simulink model "model432"  (R2014a)
settings: Solver=ode1  StartTime=0.0  StopTime=inf  FixedStep=0.002  RelTol=1e-3
PostLoadFcn:
  | qc_set_target_type(getConfigSet(bdroot, 'QUARC Default Target Configuration'));
values from neighbouring files (symbols this model uses):
  A_o = [0 1 0 0 0 0; 0 0 0 0 0 0; 0 0 0 1 0 0; 0 0 0 0 0 0; 0 0 0 0 0 1; K_3 0 0 0 0 0]    [Full_code.m]    (also in code421.m; code422.m; code431.m; code432.m)
  B_o = [0 0; 0 K_1; 0 0; K_2 0; 0 0; 0 0]    [Full_code.m]    (also in code421.m; code422.m; code431.m; code432.m)
  C_o = [1 0 0 0 0 0; 0 0 1 0 0 0; 0 0 0 0 1 0]    [Full_code.m]    (also in code421.m; code422.m; code431.m = [0 0 1 0 0 0; 0 0 0 0 1 0]; code432.m = [0 0 1 0 0 0; 0 0 0 0 1 0])
  Joystick_gain_x = 1    [Full_code.m]    (also in code13.m; code14.m; code21.m; code22.m)
  Joystick_gain_y = -1    [Full_code.m]    (also in code13.m; code14.m; code21.m; code22.m)
  K = lqr(A,B,Q,R)    [Full_code.m]    (also in code32.m; code33.m; code421.m; code422.m)
  L_o = place(transpose(A_o), transpose(C_o),poles).'    [Full_code.m]    (also in code421.m; code422.m; code431.m = place(transpose(A_o), transpose(C_o), poles).'; code432.m = place(transpose(A_o), transpose(C_o), poles).')
  P = [0 9.999999999999998;9.549869109050656 0]    [Full_code.m]    (also in code32.m = inv(C*inv(-A+B*K)*B); code33.m; code421.m = inv(C*inv(-A+B*K)*B); code422.m)
undefined symbols (not defined in the file or in its folder): HIL, qc_get_step_size
libraries: simulink_extras x6, quarc_library x4
settings Model: SimulationMode=external  ExtModeTrigDuration=5000  Creator=Rchan  LastModifiedBy=mortejan
settings SolverCC: PositivePriorityOrder=on
settings DataIOCC: SignalLoggingSaveFormat=ModelDataLogs
settings OptimizationCC: ExpressionDepthLimit=2147483647  InitFltsAndDblsToZero=on
settings DebuggingCC: SaveWithParameterizedLinksMsg=none  UnderspecifiedInitializationDetection=Classic  MultiTaskDSMMsg=warning  MultiTaskCondExecSysMsg=none  FcnCallInpInsideContextMsg=UseLocalSettings  StateNameClashWarn=warning
settings RTWCC: SystemTargetFile=quarc_win64.tlc  TemplateMakefile=quarc_default_tmf  Description=QUARC Win64 Target  ProcessScript=quarc_win64_make_rtw_hook
settings STFCustomTargetCC: CPPClassGenCompliant=on
settings GRTTargetCC: ParMdlRefBuildCompliant=off  CompOptLevelCompliant=off  CombineOutputUpdateFcns=off  MatFileLogging=off  GRTInterface=on  ExtMode=on  ExtModeMexFile=quarc_comm

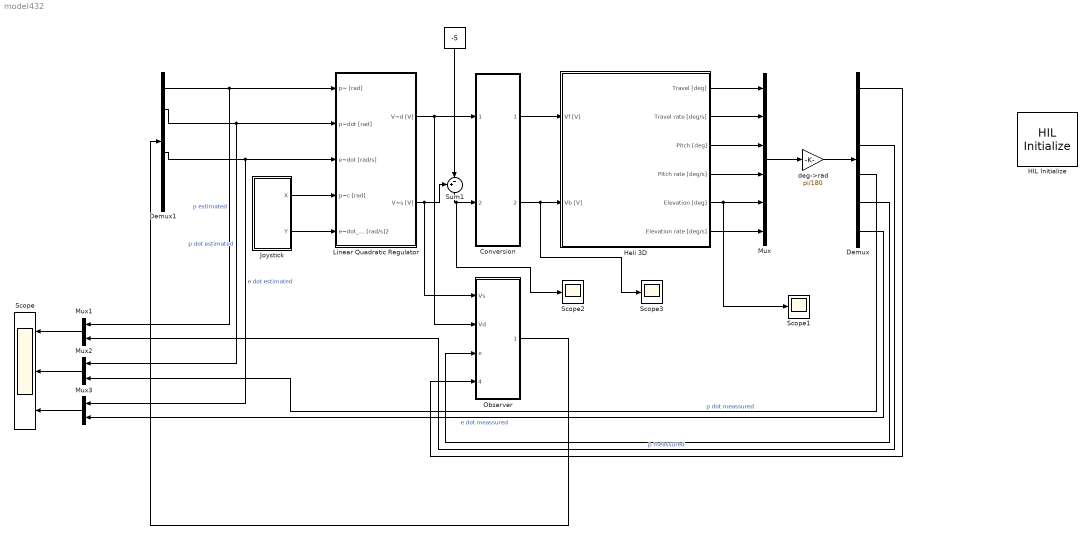
== system model432 ==
  " " : Constant  Value=-5
  Conversion : Subsystem
  Demux : Demux  Outputs=6
  Demux1 : Demux  Outputs=6
  HIL Initialize : quarc_library/Data Acquisition/Generic/Configuration/HIL Initialize  Priority=-99  object_name=HIL-1  board_type=q8_usb  board_number=0  board_options=update_rate=normal;decimation=1  exclusive=off  active=off  hardware_clocks=[0:2]  clock_modes=[]  initial_clock_frequencies=[]  set_clock_params_at_start=off  set_clock_params_at_switch_in=off  set_clock_frequencies_at_start=off  set_clock_frequencies_at_switch_in=off  analog_input_channels=[0:7]  analog_input_maximums=10  analog_input_minimums=-10  set_analog_input_params_at_start=on  set_analog_input_params_at_switch_in=off  analog_output_channels=[0:7]  analog_output_maximums=10  analog_output_minimums=-10  initial_analog_outputs=[0]  final_analog_outputs=[0]  watchdog_analog_outputs=0  set_analog_output_params_at_start=on  set_analog_output_params_at_switch_in=off  set_analog_outputs_at_start=on  set_analog_outputs_at_switch_in=off  set_analog_outputs_at_terminate=on  set_analog_outputs_at_switch_out=off  set_analog_outputs_on_watchdog=off  digital_input_channels=[]  digital_output_channels=[]  digital_output_configuration=[]  initial_digital_outputs=[1]  final_digital_outputs=[1]  watchdog_digital_outputs=[1]  set_digital_output_params_at_start=off  set_digital_output_params_at_switch_in=off  set_digital_outputs_at_start=on  set_digital_outputs_at_switch_in=off  set_digital_outputs_at_terminate=on  set_digital_outputs_at_switch_out=off  set_digital_outputs_on_watchdog=off  encoder_channels=[0:7]  quadrature=[4]  encoder_filter_frequency=[]  initial_encoder_counts=[0]  set_encoder_params_at_start=on  set_encoder_params_at_switch_in=off  set_encoder_counts_at_start=on  set_encoder_counts_at_switch_in=off  pwm_channels=[0:7]  pwm_modes=0  pwm_frequency=99.532799999999995e6/4095  pwm_configuration=[0]  pwm_alignment=[0]  pwm_polarity=[1]  pwm_leading_deadband=[0]  pwm_trailing_deadband=[0]  initial_pwm_outputs=[0]  final_pwm_outputs=[0]  watchdog_pwm_outputs=[0]  set_pwm_params_at_start=on  set_pwm_params_at_switch_in=off  set_pwm_outputs_at_start=on  set_pwm_outputs_at_switch_in=off  set_pwm_outputs_at_terminate=on  set_pwm_outputs_at_switch_out=off  set_pwm_outputs_on_watchdog=off  other_output_channels=[]  initial_other_outputs=[]  final_other_outputs=[]  watchdog_other_outputs=[]  set_other_outputs_at_start=off  set_other_outputs_at_switch_in=off  set_other_outputs_at_terminate=off  set_other_outputs_at_switch_out=off  set_other_outputs_on_watchdog=off
  Heli 3D : Subsystem
  Joystick : Subsystem
  Linear Quadratic Regulator : Subsystem
  Mux : Mux  Inputs=6
  Mux1 : Mux  Inputs=2
  Mux2 : Mux  Inputs=2
  Mux3 : Mux  Inputs=2
  Observer : Subsystem
  Scope : Scope  NumInputPorts=3
      settings: ShowLegends=on  YMin=-0.4~-1.5~-0.6  YMax=1~1.5~0.6  SaveName=ScopeData3  MaxDataPoints=10000
  Scope1 : Scope
      settings: SaveName=ScopeData4
  Scope2 : Scope
      settings: SaveName=ScopeData6
  Scope3 : Scope
      settings: SaveName=ScopeData14
  Sum1 : Sum  Inputs=+-|
  deg->rad : Gain  Gain=pi/180
  wires:
  Conversion/2(Vb [V]) -> Scope3/1, Heli 3D/2(Vb [V])
  Conversion/1(Vf [V]) -> Heli 3D/1(Vf [V])
  Heli 3D/1(Travel [deg]) -> Mux/1
  Heli 3D/2(Travel rate [deg/s]) -> Mux/2
  Heli 3D/3(Pitch [deg]) -> Mux/3
  Heli 3D/4(Pitch rate [deg/s]) -> Mux/4
  Heli 3D/5(Elevation [deg]) -> Scope1/1, Mux/5
  Heli 3D/6(Elevation rate [deg/s]) -> Mux/6
  Mux/1 -> deg->rad/1
  deg->rad/1 -> Demux/1
  Joystick/1(X) -> Linear Quadratic Regulator/4(p~c [rad])
  Joystick/2(Y) -> Linear Quadratic Regulator/5(e~dot_c [rad/s]2)
  Linear Quadratic Regulator/1(V~d [V]) -> Observer/2(Vd), Conversion/1(Vd [V])
  Linear Quadratic Regulator/2(V~s [V]) -> Observer/1(Vs), Sum1/1
  Demux/5 -> Observer/3(e)
  Demux/1 -> Observer/4(lambda)
  Observer/1(x_obs) -> Demux1/1
  Demux1/1 -> Mux1/1, Linear Quadratic Regulator/1(p~ [rad])  "p estimated"
  Demux1/2 -> Mux2/1, Linear Quadratic Regulator/2(p~dot [rad])  "p dot estimated"
  Demux1/4 -> Mux3/1, Linear Quadratic Regulator/3(e~dot [rad/s])  "e dot estimated"
  Demux/3 -> Mux1/2  "p meassured"
  Mux1/1 -> Scope/1
  Mux3/1 -> Scope/3
  Mux2/1 -> Scope/2
  Demux/4 -> Mux2/2  "p dot meassured"
  Demux/6 -> Mux3/2  "e dot meassured"
  " "/1 -> Sum1/2
  Sum1/1 -> Scope2/1, Conversion/2(Vs [V])

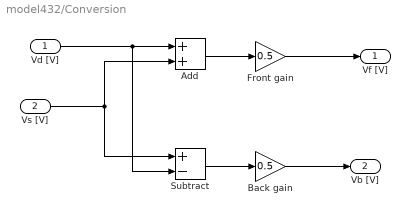
== system model432/Conversion ==
  Vd [V] : Inport
  Vs [V] : Inport  Port=2
  Add : Sum
  Back gain : Gain  Gain=0.5
  Front gain : Gain  Gain=0.5
  Subtract : Sum  Inputs=+-
  Vf [V] : Outport
  Vb [V] : Outport  Port=2
  wires:
  Vd [V]/1 -> Subtract/2, Add/1
  Vs [V]/1 -> Subtract/1, Add/2
  Subtract/1 -> Back gain/1
  Back gain/1 -> Vb [V]/1
  Add/1 -> Front gain/1
  Front gain/1 -> Vf [V]/1

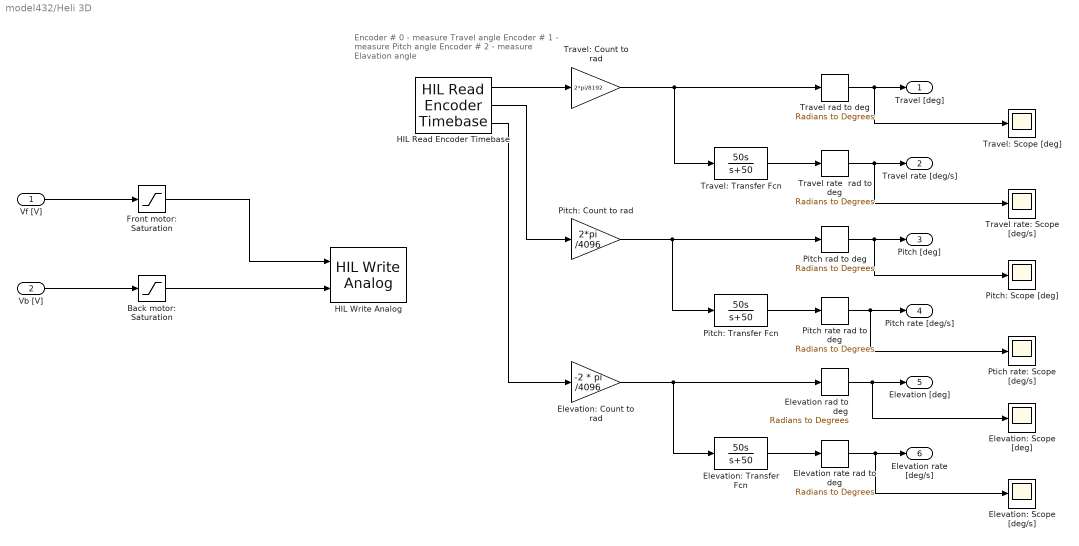
== system model432/Heli 3D ==
  note: Encoder # 0 - measure Travel angle
      | Encoder # 1 - measure Pitch angle
      | Encoder # 2 - measure Elavation angle
  Vf [V] : Inport
  Vb [V] : Inport  Port=2
  Back motor: Saturation : Saturate  UpperLimit=5  LowerLimit=-5
  Elevation rad to deg : simulink_extras/Transformations/Radians to Degrees
  Elevation rate rad to deg : simulink_extras/Transformations/Radians to Degrees
  Elevation: Count to rad : Gain  Gain=-2 * pi /4096
  Elevation: Scope [deg/s] : Scope
      settings: YMin=-15  YMax=15  SaveName=ScopeData13
  Elevation: Scope [deg] : Scope
      settings: YMin=-15  YMax=15  SaveName=ScopeData12
  Elevation: Transfer Fcn : TransferFcn  Numerator=[50 0]  Denominator=[1 50]
  Front motor: Saturation : Saturate  UpperLimit=5  LowerLimit=-5
  HIL Read Encoder Timebase : quarc_library/Data Acquisition/Generic/Timebases/HIL Read Encoder Timebase  object_name=HIL-1  clock=0  channels=[0:2]  samples_in_buffer=max(ceil(1/qc_get_step_size), 1)  active=on  vector_output=off  data_type_mode=Inherit via back propagation  data_type=double
  HIL Write Analog : quarc_library/Data Acquisition/Generic/Immediate I//O/HIL Write Analog  object_name=HIL-1  channels=[0:1]  sample_time=-1  active=off  vector_input=off
  Pitch rad to deg : simulink_extras/Transformations/Radians to Degrees
  Pitch rate rad to deg : simulink_extras/Transformations/Radians to Degrees
  Pitch: Count to rad : Gain  Gain=2*pi /4096
  Pitch: Scope [deg] : Scope
      settings: YMin=-15  YMax=15  SaveName=ScopeData10
  Pitch: Transfer Fcn : TransferFcn  Numerator=[50 0]  Denominator=[1 50]
  Ptich rate: Scope [deg/s] : Scope
      settings: YMin=-15  YMax=15  SaveName=ScopeData11
  Travel rad to deg : simulink_extras/Transformations/Radians to Degrees
  Travel rate  rad to deg : simulink_extras/Transformations/Radians to Degrees
  Travel rate: Scope [deg/s] : Scope
      settings: YMin=-15  YMax=15  SaveName=ScopeData9
  Travel: Count to rad : Gain  Gain=2*pi/8192
  Travel: Scope [deg] : Scope
      settings: YMin=-15  YMax=15  SaveName=ScopeData8
  Travel: Transfer Fcn : TransferFcn  Numerator=[50 0]  Denominator=[1 50]
  Travel [deg] : Outport
  Travel rate [deg/s] : Outport  Port=2
  Pitch [deg] : Outport  Port=3
  Pitch rate [deg/s] : Outport  Port=4
  Elevation [deg] : Outport  Port=5
  Elevation rate [deg/s] : Outport  Port=6
  wires:
  HIL Read Encoder Timebase/1 -> Travel: Count to rad/1
  HIL Read Encoder Timebase/2 -> Pitch: Count to rad/1
  HIL Read Encoder Timebase/3 -> Elevation: Count to rad/1
  Travel: Count to rad/1 -> Travel: Transfer Fcn/1, Travel rad to deg/1
  Travel: Transfer Fcn/1 -> Travel rate  rad to deg/1
  Pitch: Count to rad/1 -> Pitch: Transfer Fcn/1, Pitch rad to deg/1
  Pitch: Transfer Fcn/1 -> Pitch rate rad to deg/1
  Elevation: Count to rad/1 -> Elevation: Transfer Fcn/1, Elevation rad to deg/1
  Elevation: Transfer Fcn/1 -> Elevation rate rad to deg/1
  Travel rad to deg/1 -> Travel: Scope [deg]/1, Travel [deg]/1
  Travel rate  rad to deg/1 -> Travel rate: Scope [deg/s]/1, Travel rate [deg/s]/1
  Pitch rad to deg/1 -> Pitch: Scope [deg]/1, Pitch [deg]/1
  Pitch rate rad to deg/1 -> Ptich rate: Scope [deg/s]/1, Pitch rate [deg/s]/1
  Elevation rad to deg/1 -> Elevation: Scope [deg]/1, Elevation [deg]/1
  Elevation rate rad to deg/1 -> Elevation: Scope [deg/s]/1, Elevation rate [deg/s]/1
  Vf [V]/1 -> Front motor: Saturation/1
  Vb [V]/1 -> Back motor: Saturation/1
  Front motor: Saturation/1 -> HIL Write Analog/1
  Back motor: Saturation/1 -> HIL Write Analog/2

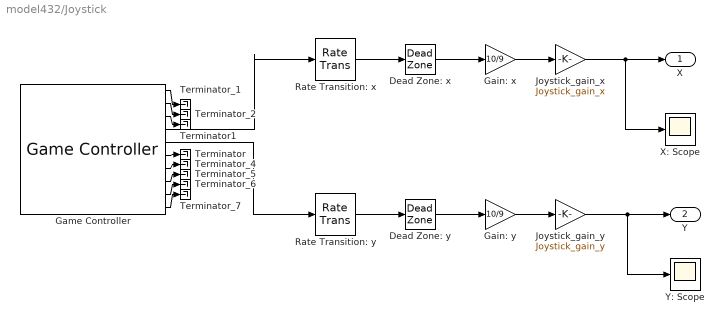
== system model432/Joystick ==
  Dead Zone: x : DeadZone  LowerValue=-0.1  UpperValue=0.1  SaturateOnIntegerOverflow=on
  Dead Zone: y : DeadZone  LowerValue=-0.1  UpperValue=0.1  SaturateOnIntegerOverflow=on
  Gain: x : Gain  Gain=10/9
  Gain: y : Gain  Gain=10/9
  Game Controller : quarc_library/Devices/Peripherals/Target/Game Controller  controller=1  buffer_size=12  deadzone=[]  saturation=[]  sample_time=max(qc_get_step_size, 0.01)  auto_center=off  enabled=on
  Joystick_gain_x : Gain  Gain=Joystick_gain_x
  Joystick_gain_y : Gain  Gain=Joystick_gain_y
  Rate Transition: x : RateTransition
  Rate Transition: y : RateTransition
  Terminator : Terminator
  Terminator1 : Terminator
  Terminator_{1..2,4..7} (6 alike) : Terminator
  X: Scope : Scope
      settings: YMin=-1  YMax=1  SaveName=ScopeData7
  Y: Scope : Scope
      settings: YMin=-10  YMax=10  SaveName=ScopeData5
  X : Outport
  Y : Outport  Port=2
  wires:
  Rate Transition: y/1 -> Dead Zone: y/1
  Rate Transition: x/1 -> Dead Zone: x/1
  Game Controller/5 -> Rate Transition: y/1
  Game Controller/4 -> Rate Transition: x/1
  Game Controller/1 -> Terminator_1/1
  Game Controller/2 -> Terminator_2/1
  Game Controller/7 -> Terminator_4/1
  Game Controller/8 -> Terminator_5/1
  Game Controller/9 -> Terminator_6/1
  Game Controller/10 -> Terminator_7/1
  Game Controller/3 -> Terminator1/1
  Game Controller/6 -> Terminator/1
  Dead Zone: x/1 -> Gain: x/1
  Dead Zone: y/1 -> Gain: y/1
  Gain: x/1 -> Joystick_gain_x/1
  Gain: y/1 -> Joystick_gain_y/1
  Joystick_gain_x/1 -> X/1, X: Scope/1
  Joystick_gain_y/1 -> Y: Scope/1, Y/1

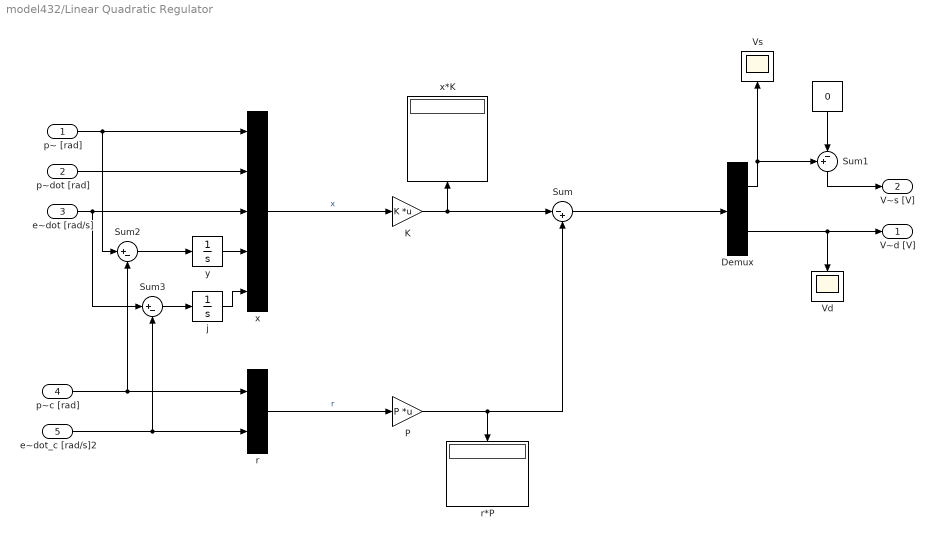
== system model432/Linear Quadratic Regulator ==
  p~ [rad] : Inport
  p~dot [rad] : Inport  Port=2
  e~dot [rad/s] : Inport  Port=3
  p~c [rad] : Inport  Port=4
  e~dot_c [rad/s]2 : Inport  Port=5
  " " : Constant  Value=0
  Demux : Demux  Outputs=2
  K : Gain  Gain=K  Multiplication=Matrix(K*u)
  P : Gain  Gain=P  Multiplication=Matrix(K*u)
  Sum : Sum  Inputs=|-+
  Sum1 : Sum  Inputs=+-|
  Sum2 : Sum  Inputs=|+-
  Sum3 : Sum  Inputs=|+-
  Vd : Scope
  Vs : Scope
      settings: YMin=-6  YMax=9
  j : Integrator
  r : Concatenate
  r*P : Display
  x : Concatenate  NumInputs=5
  x*K : Display
  y : Integrator
  V~d [V] : Outport  InitialOutput=0
  V~s [V] : Outport  Port=2  InitialOutput=0
  wires:
  p~c [rad]/1 -> r/1, Sum2/2
  p~ [rad]/1 -> Sum2/1, x/1
  p~dot [rad]/1 -> x/2
  e~dot [rad/s]/1 -> Sum3/1, x/3
  e~dot_c [rad/s]2/1 -> Sum3/2, r/2
  r/1 -> P/1  "r"
  x/1 -> K/1  "x"
  K/1 -> Sum/1, x*K/1
  P/1 -> Sum/2, r*P/1
  Sum/1 -> Demux/1
  Demux/2 -> V~d [V]/1, Vd/1
  Demux/1 -> Sum1/1, Vs/1
  Sum1/1 -> V~s [V]/1
  " "/1 -> Sum1/2
  Sum2/1 -> y/1
  Sum3/1 -> j/1
  y/1 -> x/4
  j/1 -> x/5

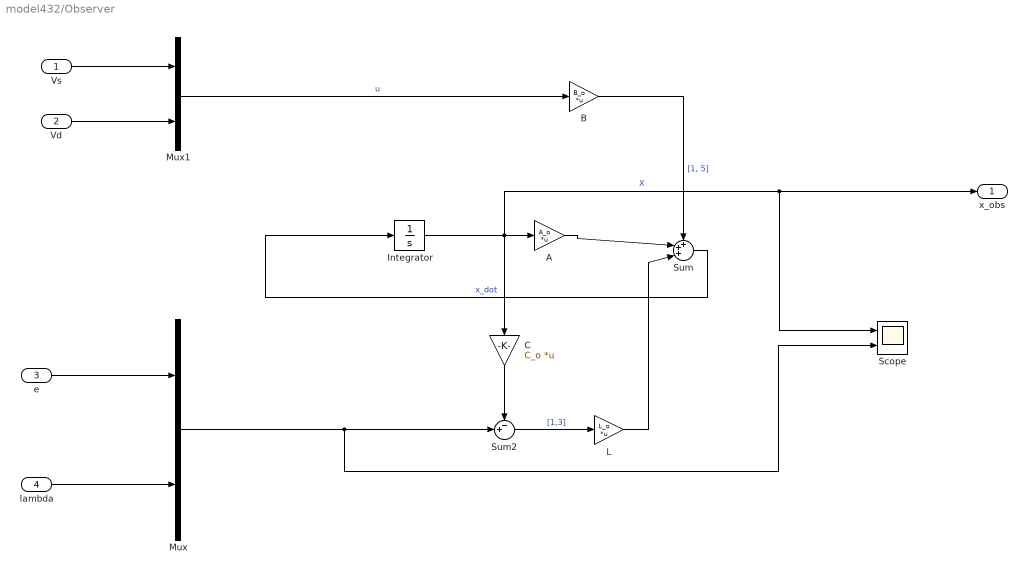
== system model432/Observer ==
  Vs : Inport
  Vd : Inport  Port=2
  e : Inport  Port=3
  lambda : Inport  Port=4
  A : Gain  Gain=A_o  Multiplication=Matrix(K*u)
  B : Gain  Gain=B_o  Multiplication=Matrix(K*u)
  C : Gain  Gain=C_o  Multiplication=Matrix(K*u)
  Integrator : Integrator
  L : Gain  Gain=L_o  Multiplication=Matrix(K*u)
  Mux : Mux  Inputs=2
  Mux1 : Mux  Inputs=2
  Scope : Scope  NumInputPorts=2
      settings: YMin=-35~-35  YMax=5~5  SaveName=ScopeData2
  Sum : Sum  Inputs=+++|
  Sum2 : Sum  Inputs=-+|
  x_obs : Outport
  wires:
  Sum2/1 -> L/1  "[1,3]"
  Vs/1 -> Mux1/1
  Vd/1 -> Mux1/2
  Mux1/1 -> B/1  "u"
  C/1 -> Sum2/1
  Sum/1 -> Integrator/1  "x_dot"
  L/1 -> Sum/3
  A/1 -> Sum/2
  B/1 -> Sum/1  "[1, 5]"
  lambda/1 -> Mux/2
  Integrator/1 -> Scope/1, x_obs/1, C/1, A/1  "X"
  Mux/1 -> Scope/2, Sum2/2
  e/1 -> Mux/1
